simulink model "StateMachineModel"  (R2021b)
settings: Solver=VariableStepAuto  StartTime=0.0  StopTime=1.0  RelTol=1e-3
model workspace (MATLAB code in the model file):
  | addpath model
  | addpath utils
libraries: simulink x1
settings Model: Creator=raquelgrillo  LastModifiedBy=andrerangel

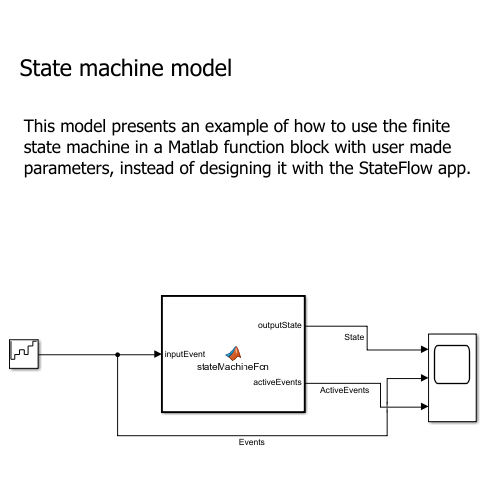
[thumbnail: Simulink's stored preview of the top-level diagram]
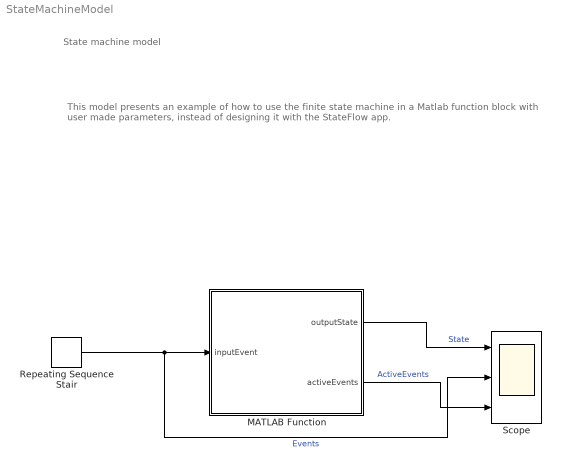
== system StateMachineModel ==
  note: State machine model
  note: This model presents an example of how to use the finite state machine in a Matlab function block with user made parameters, instead of designing it with the StateFlow app.
  MATLAB Function : MATLAB Function  TreatAsAtomicUnit=on
  Repeating Sequence Stair : simulink/Sources/Repeating Sequence Stair  OutValues=[1 2 3 2 4 5]  tsamp=-1  OutMin=[]  OutMax=[]  OutDataTypeStr=double  OutputDataTypeScalingMode=double  OutDataType=fixdt(0,8)  ConRadixGroup=Best Precision: Vector-wise  OutScaling=2^-12
  Scope : Scope  NumInputPorts=3
  wires:
  MATLAB Function/1(outputState) -> Scope/1  "State"
  Repeating Sequence Stair/1 -> Scope/2, MATLAB Function/1(inputEvent)  "Events"
  MATLAB Function/2(activeEvents) -> Scope/3  "ActiveEvents"

== matlab function StateMachineModel/MATLAB Function ==
  data: inputEvent input; outputState output size=[1 1]; activeEvents output
function [outputState, activeEvents]  = stateMachineFcn(inputEvent)
% Example of a State Machine with 3 states.
persistent stateMachine

if (isempty(stateMachine))
    
    % Create the states with the State Class.
    s0 = State(0, 's0', [1,0,1,1,1]);
    s1 = State(1, 's1', [1,1,0,1,1]);
    s2 = State(2, 's2', [1,0,1,1,1]);

    % Group it in a cell array.
    statesArray = {s0, s1, s2};

    % Transitions matrix where each line represents a transition: 
    % event 2 makes a transitions from state 0 to 2 is represented as 
    % [0 2 1]
    transitions = [0, 1 0; 0, 2, 1; 1, 3, 0; 1, 4, 2; 2, 5, 1; 2, 1, 0];

    % Array with the number of the events.
    eventsArray = [1 2 3 4 5];
    stateMachine = StateMachine(statesArray, transitions, eventsArray);
end

stateMachine.inputEvent = inputEvent;
outputState = stateMachine.currentState.number;

activeEvents = stateMachine.currentState.activeEvents;
